simulink model "P3P_Grunert"  (R2023b)
settings: Solver=FixedStepDiscrete  StartTime=0.0  StopTime=0  RelTol=1e-3
values from neighbouring files (symbols this model uses):
  checkerSize = [5, 8]    [P3P_processVideo.m]
  checkerSquareLength = 31    [P3P_processVideo.m]
  I_current = I_allFrames(:,:,q)    [P3P_processVideo.m]
  K = [1107 0 960; 0 1107 540; 0 0 1]    [P3P_processVideo.m]
  x_pnts_i = round(x_pnts_i)    [P3P_processVideo.m]
undefined symbols (not defined in the file or in its folder): gray, Rec, SDTV, X_pnts_w
libraries: dspinverses x4, dspmathops x4, visiontextngfix x4, visionconversions x1, visionanalysis x1, dspvision x1, visionsources x1
(part 1 of 2)
settings Model: Creator=The MathWorks, Inc.  LastModifiedBy=alyss
settings DebuggingCC: ParameterPrecisionLossMsg=none  UnconnectedInputMsg=warning  UnconnectedOutputMsg=warning  UnconnectedLineMsg=warning  IntegerSaturationMsg=none
settings ModelReferenceCC: EnableRefExpFcnMdlSchedulingChecks=on
settings RTWCC: DLArmComputeVersion=19.05

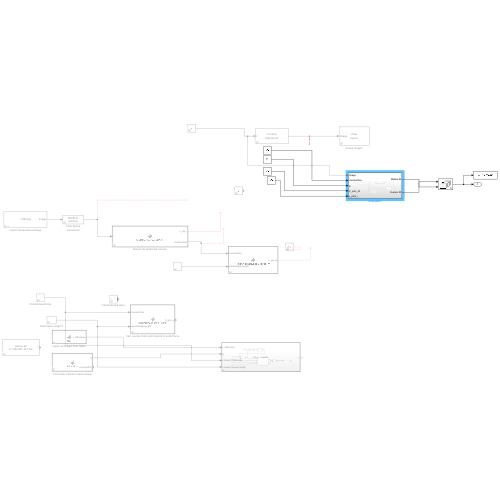
[thumbnail: Simulink's stored preview of the top-level diagram]
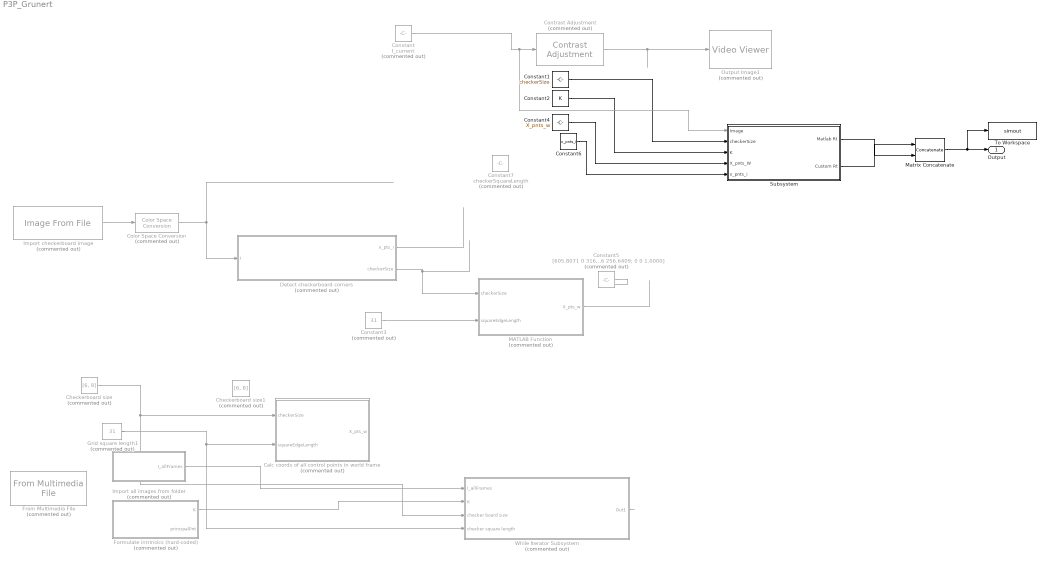
== system P3P_Grunert ==
  Calc coords of all control points in world frame : MATLAB Function  Commented=on  TreatAsAtomicUnit=on
  Checkerboard size : Constant  Commented=on  Value=[6, 8]
  Checkerboard size1 : Constant  Commented=on  Value=[6, 8]
  Color Space Conversion : visionconversions/Color Space  Conversion  Commented=on  conversion=Obsolete  conversionActive=R'G'B' to intensity  wp_str=D65  rec=Rec. 601 (SDTV)  sys=1125/60/2:1  imagePorts=One multidimensional signal
  Constant : Constant  Commented=on  Value=I_current
  Constant1 : Constant  Value=checkerSize
  Constant2 : Constant  Value=K
  Constant3 : Constant  Commented=on  Value=31
  Constant4 : Constant  Value=X_pnts_w
  Constant5 : Constant  Commented=on  Value=[605.8071 0 316.6903; 0 608.4646 256.6409; 0 0 1.0000]
  Constant6 : Constant  Value=x_pnts_i
  Constant7 : Constant  Commented=on  Value=checkerSquareLength
  Contrast Adjustment : visionanalysis/Contrast Adjustment  Commented=on  methodInputRange=Full input data range [min max]  rangeIn=[0 255]  fracSaturate=[1 1]  isBinNum=on  binNum=256  methodOutputRange=Full data type range  rangeOut=[0 255]  roundingMode=Floor  overflowMode=off  prod1Mode=Binary point scaling  prod1WordLength=32  prod1FracLength=16  prod2Mode=Binary point scaling  prod2WordLength=32  prod2FracLength=16
  Detect checkerboard corners : MATLAB Function  Commented=on  TreatAsAtomicUnit=on
  Formulate intrinsics (hard-coded) : MATLAB Function  Commented=on  TreatAsAtomicUnit=on
  From Multimedia File : dspvision/From Multimedia File  Commented=on  inputFilename=vipmen.avi  readRange=[1 Inf]  loop=on  numPlays=1  outputStreams=Video only  videoDataType=single  audioDataType=int16  inheritSampleTime=on  userDefinedSampleTime=1/30  noAudioOutput=off  isIntensityVideo=off  fourcc=Intensity  colorVideoFormat=One multidimensional signal  outputEOF=off  dataOrg=Column-major  audioFrameSize=1024  computeAudioFrameSize=off  outSamplingMode=Sample based
      settings: LibrarySourceBlock=visionsources/From Multimedia File
  Grid square length1 : Constant  Commented=on  Value=31
  Import all images from folder : MATLAB Function  Commented=on  TreatAsAtomicUnit=on
  Import checkerboard image : visionsources/Image From File  Tag=vipblks_nd  Commented=on  FileName=C:\Users\alyss\OneDrive - University of Cape Town\Code\MATLAB\PnP\Verification\-0160.jpg  Ts=inf  imagePorts=One multidimensional signal  OutPortLabels=R|G|B  ImageDataType=Inherit from input image  sdImageDataType=uint(8)  Signed=on  WordLength=16  FractionLengthMode=User-defined  FractionLength=15
  MATLAB Function : MATLAB Function  Commented=on  TreatAsAtomicUnit=on
  Matrix Concatenate : Concatenate  Mode=Multidimensional array  ConcatenateDimension=3
  Output Image1 : VideoViewer  Commented=on  colormapValue=gray(256)  FigPos=[1727 991 1362 617]
  Subsystem : Subsystem
  To Workspace : ToWorkspace  VariableName=simout  SampleTime=-1
  While Iterator Subsystem : Subsystem  Commented=on  TreatAsAtomicUnit=on
  Output : Outport
  wires:
  Import checkerboard image/1 -> Color Space Conversion/1
  Subsystem/1(Matlab Rt) -> Matrix Concatenate/2
  Subsystem/2(Custom Rt) -> Matrix Concatenate/1
  Matrix Concatenate/1 -> To Workspace/1, Output/1
  Formulate intrinsics (hard-coded)/1(K) -> While Iterator Subsystem/2(K)
  Grid square length1/1 -> Calc coords of all control points in world frame/2(squareEdgeLength), While Iterator Subsystem/4(checker square length)
  While Iterator Subsystem/1(Out1) -> ?
  Import all images from folder/1(I_allFrames) -> While Iterator Subsystem/1(I_allFrames)
  Constant3/1 -> MATLAB Function/2(squareEdgeLength)
  Checkerboard size/1 -> While Iterator Subsystem/3(checker board size), Calc coords of all control points in world frame/1(checkerSize)
  Constant4/1 -> Subsystem/4(X_pnts_W)
  Contrast Adjustment/1 -> Output Image1/1
  Constant1/1 -> Subsystem/2(checkerSize)
  Constant2/1 -> Subsystem/3(K)
  Color Space Conversion/1 -> Detect checkerboard corners/1(I)
  Constant/1 -> Subsystem/1(Image), Contrast Adjustment/1
  Constant6/1 -> Subsystem/5(x_pnts_i)
  Detect checkerboard corners/1(x_pts_i) -> ?
  Detect checkerboard corners/2(checkerSize) -> MATLAB Function/1(checkerSize)
  Constant5/1 -> ?
  MATLAB Function/1(X_pts_w) -> ?

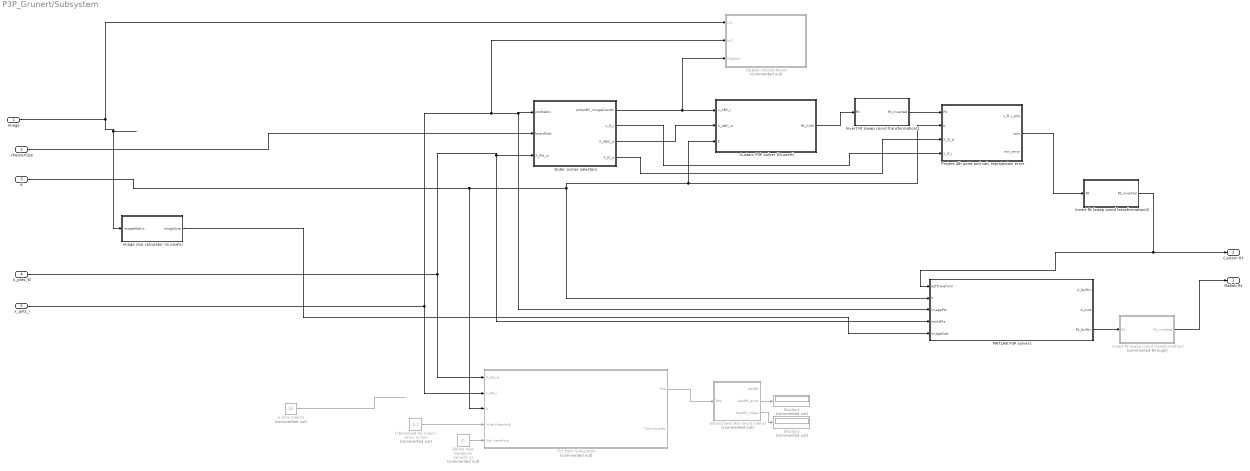
== system P3P_Grunert/Subsystem ==
  Image : Inport
  checkerSize : Inport  Port=2
  K : Inport  Port=3
  X_pnts_W : Inport  Port=4
  x_pnts_i : Inport  Port=5
  Custom P3P solver (Grunert) : Subsystem
  Define max iterations : Constant  Commented=on  Value=zeros(5,1)
  Display checkerboard : Subsystem  Commented=on
  Display4 : Display  Commented=on
  Display5 : Display  Commented=on
  Extract best Rte (most inliers) : MATLAB Function  Commented=on  TreatAsAtomicUnit=on
  For Each Subsystem : Subsystem  Commented=on  TreatAsAtomicUnit=on
  Image size calculator (in pixels) : MATLAB Function  TreatAsAtomicUnit=on
  Invert Rt (swap coord transformation) : MATLAB Function  Commented=through  TreatAsAtomicUnit=on
  Invert Rt (swap coord transformation)1 : MATLAB Function  TreatAsAtomicUnit=on
  Invert Rt (swap coord transformation)2 : MATLAB Function  TreatAsAtomicUnit=on
  MATLAB P3P solver1 : MATLAB Function  TreatAsAtomicUnit=on
  Outer corner selectors : Subsystem
  Project 4th point and calc reprojection error : MATLAB Function  TreatAsAtomicUnit=on
  n (min inliers) : Constant  Commented=on  Value=25
  t (threshold for inlier) - error in mm : Constant  Commented=on  Value=0.7
  Matlab Rt : Outport
  Custom Rt : Outport  Port=2
  wires:
  n (min inliers)/1 -> ?
  t (threshold for inlier) - error in mm/1 -> For Each Subsystem/4(Inlier threshold)
  Outer corner selectors/4(X_D_w) -> Project 4th point and calc reprojection error/3(X_D_w)
  Outer corner selectors/2(x_D_i) -> Project 4th point and calc reprojection error/4(x_D_i)
  x_pnts_i/1 -> MATLAB P3P solver1/3(imagePts), Outer corner selectors/1(pntMatrix), Display checkerboard/2(In2), For Each Subsystem/2(x_pts_i)
  Extract best Rte (most inliers)/2(bestRt_error) -> Display4/1
  Image/1 -> Image size calculator (in pixels)/1(imageMatrix), Display checkerboard/1(In1)
  X_pnts_W/1 -> MATLAB P3P solver1/4(worldPts), Outer corner selectors/3(X_Pts_w), For Each Subsystem/1(X_pts_w)
  For Each Subsystem/1(Rte) -> Extract best Rte (most inliers)/1(Rte)
  Outer corner selectors/3(X_ABC_w) -> Custom P3P solver (Grunert)/2(X_ABC_w)
  Extract best Rte (most inliers)/3(bestRt_inliers) -> Display5/1
  Image size calculator (in pixels)/1(imageSize) -> MATLAB P3P solver1/5(imageSize)
  K/1 -> For Each Subsystem/3(K), Project 4th point and calc reprojection error/2(K), Custom P3P solver (Grunert)/3(K), MATLAB P3P solver1/2(K)
  Define max iterations/1 -> For Each Subsystem/5(Vec iterations)
  Outer corner selectors/1(pntsABC_imageCoords) -> Display checkerboard/3(Outport), Custom P3P solver (Grunert)/1(x_ABC_i)
  checkerSize/1 -> Outer corner selectors/2(boardSize)
  MATLAB P3P solver1/3(Rt_builtin) -> Invert Rt (swap coord transformation)/1(Rt)
  Invert Rt (swap coord transformation)/1(Rt_inverted) -> Matlab Rt/1
  Invert Rt (swap coord transformation)2/1(Rt_inverted) -> MATLAB P3P solver1/1(estTransform), Custom Rt/1
  Custom P3P solver (Grunert)/1(Rt_C2W) -> Invert Rt (swap coord transformation)1/1(Rt)
  Invert Rt (swap coord transformation)1/1(Rt_inverted) -> Project 4th point and calc reprojection error/1(Rt)
  Project 4th point and calc reprojection error/2(soln) -> Invert Rt (swap coord transformation)2/1(Rt)

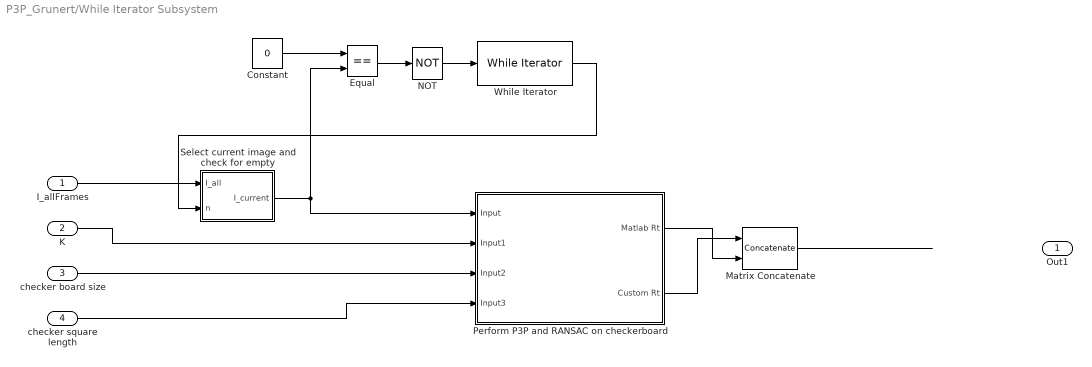
== system P3P_Grunert/While Iterator Subsystem ==
  I_allFrames : Inport
  K : Inport  Port=2
  checker board size : Inport  Port=3
  checker square length : Inport  Port=4
  Constant : Constant  Value=0
  Equal : RelationalOperator  Operator===  OutDataTypeStr=boolean  RndMeth=Simplest  InputSameDT=off
  Matrix Concatenate : Concatenate  Mode=Multidimensional array  ConcatenateDimension=3
  NOT : Logic  Operator=NOT  IconShape=distinctive  AllPortsSameDT=off  OutDataTypeStr=boolean
  Perform P3P and RANSAC on checkerboard : Subsystem  mask{intensityMatrix=[0 0; 0 0], checkerSize=[0, 0], K=[0 0 0; 0 0 0; 0 0 0], checkerSquareEdgeLength=0}
      mask prompts: intensityMatrix "2D matrix of pixel intensity values."; checkerSize "Number of squares in the checkerboard to be detected, specified as a 1D array [height, width]."; K "Camera intrinsic matrix, 3x3."; checkerSquareEdgeLength "Length of edge of one square in mm."
  Select current image and check for empty : MATLAB Function  TreatAsAtomicUnit=on
  While Iterator : WhileIterator  MaxIters=100  WhileBlockType=do-while  ShowIterationPort=on  OutputDataType=int16
  Out1 : Outport
  wires:
  I_allFrames/1 -> Select current image and check for empty/1(I_all)
  While Iterator/1 -> Select current image and check for empty/2(n)
  Constant/1 -> Equal/1
  NOT/1 -> While Iterator/1
  Equal/1 -> NOT/1
  Select current image and check for empty/1(I_current) -> Perform P3P and RANSAC on checkerboard/1(Input), Equal/2
  Matrix Concatenate/1 -> ?
  Perform P3P and RANSAC on checkerboard/2(Custom Rt) -> Matrix Concatenate/1
  K/1 -> Perform P3P and RANSAC on checkerboard/2(Input1)
  Perform P3P and RANSAC on checkerboard/1(Matlab Rt) -> Matrix Concatenate/2
  checker square length/1 -> Perform P3P and RANSAC on checkerboard/4(Input3)
  checker board size/1 -> Perform P3P and RANSAC on checkerboard/3(Input2)

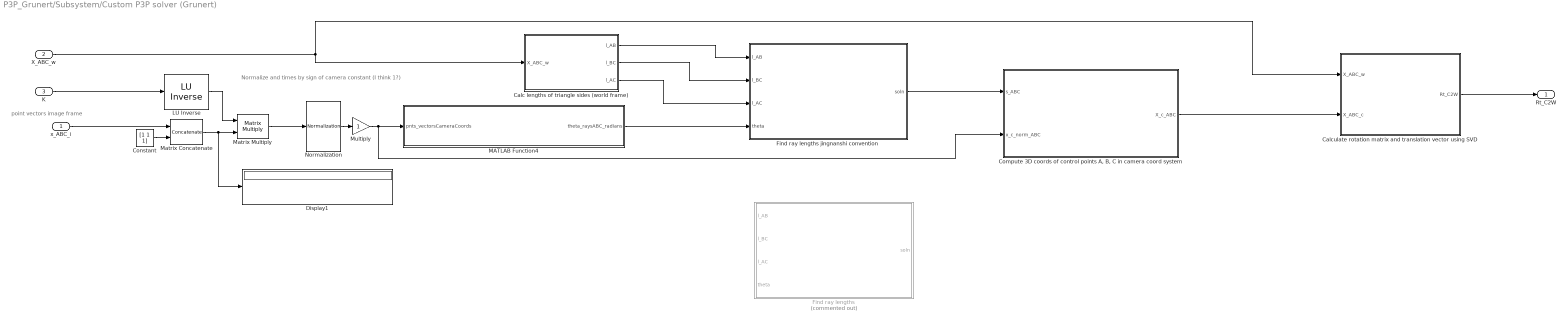
== system P3P_Grunert/Subsystem/Custom P3P solver (Grunert) ==
  note: point vectors image frame
  note: Normalize and times by sign of camera constant (I think 1?)
  x_ABC_i : Inport
  X_ABC_w : Inport  Port=2
  K : Inport  Port=3
  " LU Inverse" : dspinverses/ LU Inverse
  Calc lengths of triangle sides (world frame) : MATLAB Function  TreatAsAtomicUnit=on
  Calculate rotation matrix and translation vector using SVD : MATLAB Function  TreatAsAtomicUnit=on
  "Compute 3D coords of control points A, B, C in camera coord system" : MATLAB Function  TreatAsAtomicUnit=on
  Constant : Constant  Value=[1 1 1]  VectorParams1D=off
  Display1 : Display
  Find ray lengths : MATLAB Function  Commented=on  TreatAsAtomicUnit=on
  Find ray lengths jingnanshi convention : MATLAB Function  TreatAsAtomicUnit=on
  MATLAB Function4 : MATLAB Function  TreatAsAtomicUnit=on
  Matrix Concatenate : Concatenate  Mode=Multidimensional array
  Matrix Multiply : Product  Multiplication=Matrix(*)
  Multiply : Gain
  Normalization : dspmathops/Normalization  NormType=2-norm  Bias=1e-10  NormOver=Each column  Dimension=1  roundingMode=Floor  overflowMode=off  accumDataTypeStr=Inherit: Same as product output  accumLastDataTypeStr=Inherit: Same as product output  outputDataTypeStr=Inherit: Same as product output  outputMin=[]  outputMax=[]  outputLastDataTypeStr=Inherit: Same as product output
  Rt_C2W : Outport
  wires:
  Multiply/1 -> "Compute 3D coords of control points A, B, C in camera coord system"/2(x_c_norm_ABC), MATLAB Function4/1(pnts_vectorsCameraCoords)
  Normalization/1 -> Multiply/1
  MATLAB Function4/1(theta_raysABC_radians) -> Find ray lengths jingnanshi convention/4(theta)
  "Compute 3D coords of control points A, B, C in camera coord system"/1(X_c_ABC) -> Calculate rotation matrix and translation vector using SVD/2(X_ABC_c)
  X_ABC_w/1 -> Calculate rotation matrix and translation vector using SVD/1(X_ABC_w), Calc lengths of triangle sides (world frame)/1(X_ABC_w)
  Calc lengths of triangle sides (world frame)/3(l_AC) -> Find ray lengths jingnanshi convention/3(l_AC)
  Calc lengths of triangle sides (world frame)/1(l_AB) -> Find ray lengths jingnanshi convention/1(l_AB)
  Calc lengths of triangle sides (world frame)/2(l_BC) -> Find ray lengths jingnanshi convention/2(l_BC)
  K/1 -> " LU Inverse"/1
  Find ray lengths jingnanshi convention/1(soln) -> "Compute 3D coords of control points A, B, C in camera coord system"/1(s_ABC)
  x_ABC_i/1 -> Matrix Concatenate/1
  Matrix Concatenate/1 -> Display1/1, Matrix Multiply/2
  " LU Inverse"/1 -> Matrix Multiply/1
  Matrix Multiply/1 -> Normalization/1
  Constant/1 -> Matrix Concatenate/2
  Calculate rotation matrix and translation vector using SVD/1(Rt_C2W) -> Rt_C2W/1

== system P3P_Grunert/Subsystem/Display checkerboard ==
  In1 : Inport
  In2 : Inport  Port=2
  Outport : Inport  Port=3
  Data Type Conversion : DataTypeConversion  OutDataTypeStr=int16  SaturateOnIntegerOverflow=off  RndMeth=Floor
  Data Type Conversion1 : DataTypeConversion  OutDataTypeStr=int16  SaturateOnIntegerOverflow=off  RndMeth=Floor
  Draw All Detected Corners1 : visiontextngfix/Draw Markers  shape=Circle  size=4  fill=on  fillClrSource=Specify via dialog  display=User-specified value  intensity=200  color=250  opacity=0.6  viewport=Entire image  antialiasing=off  inType=Obsolete  imagePorts=One multidimensional signal  roundingMode=Floor  overflowMode=off  memoryMode=Specify word length  memoryWordLength=16  memoryFracLength=15  prodOutputMode=Binary point scaling  prodOutputWordLength=32  prodOutputFracLength=14
  Insert Text : visiontextngfix/Insert Text  inputType=Obsolete  theText='%s'  getTextLocFrom=Input port  textLoc=[100 100]  getTextColorFrom=Specify via dialog  textColor=[0 255 0]  getTextIntensityFrom=Specify via dialog  textIntensity=1  getTextOpacityFrom=Specify via dialog  textOpacity=1.0  dummyVar2=0  dummyVar3=0  dummyVar4=0  imagePorts=One multidimensional signal  isInputTransposed=off  fontFace=LucidaSansRegular  dummyVar1=0  blockFontSize=60  antiAliased=on
  Output Image1 : VideoViewer  colormapValue=gray(256)  FigPos=[2 725 1362 615]
  Specify text variables : Constant  Value=uint8(['A' 0 'B' 0 'C'])
  Transpose : Math  Operator=transpose
  wires:
  Data Type Conversion/1 -> Draw All Detected Corners1/2
  Draw All Detected Corners1/1 -> Insert Text/1
  Specify text variables/1 -> Insert Text/2
  Transpose/1 -> Insert Text/3
  In1/1 -> Draw All Detected Corners1/1
  Insert Text/1 -> Output Image1/1
  Data Type Conversion1/1 -> Transpose/1
  Outport/1 -> Data Type Conversion1/1
  In2/1 -> Data Type Conversion/1

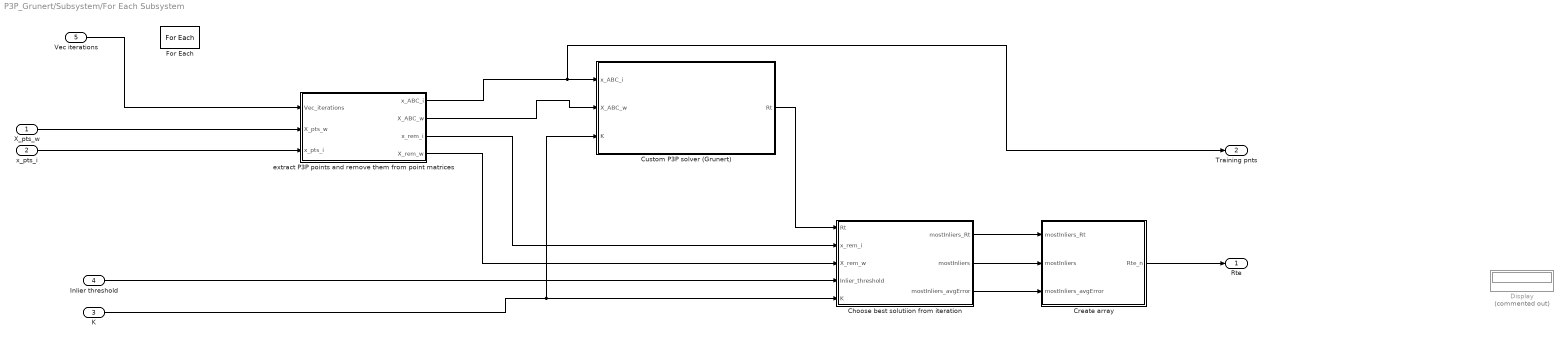
== system P3P_Grunert/Subsystem/For Each Subsystem ==
  X_pts_w : Inport
  x_pts_i : Inport  Port=2
  K : Inport  Port=3
  Inlier threshold : Inport  Port=4
  Vec iterations : Inport  Port=5  Partition=on  PartitionDimension=1  PartitionWidth=1  PartitionOffset=0
  Choose best solutiion from iteration : MATLAB Function  TreatAsAtomicUnit=on
  Create array : MATLAB Function  TreatAsAtomicUnit=on
  Custom P3P solver (Grunert) : Subsystem
  Display : Display  Commented=on
  For Each : ForEach  DisableCoverage=on
  extract P3P points and remove them from point matrices : MATLAB Function  TreatAsAtomicUnit=on
  Rte : Outport  ConcatenationDimension=3
  Training pnts : Outport  Port=2  ConcatenationDimension=2
  wires:
  Create array/1(Rte_n) -> Rte/1
  K/1 -> Custom P3P solver (Grunert)/3(K), Choose best solutiion from iteration/5(K)
  Choose best solutiion from iteration/2(mostInliers) -> Create array/2(mostInliers)
  Choose best solutiion from iteration/1(mostInliers_Rt) -> Create array/1(mostInliers_Rt)
  Inlier threshold/1 -> Choose best solutiion from iteration/4(Inlier_threshold)
  Custom P3P solver (Grunert)/1(Rt) -> Choose best solutiion from iteration/1(Rt)
  x_pts_i/1 -> extract P3P points and remove them from point matrices/3(x_pts_i)
  extract P3P points and remove them from point matrices/4(X_rem_w) -> Choose best solutiion from iteration/3(X_rem_w)
  extract P3P points and remove them from point matrices/1(x_ABC_i) -> Training pnts/1, Custom P3P solver (Grunert)/1(x_ABC_i)
  X_pts_w/1 -> extract P3P points and remove them from point matrices/2(X_pts_w)
  extract P3P points and remove them from point matrices/2(X_ABC_w) -> Custom P3P solver (Grunert)/2(X_ABC_w)
  extract P3P points and remove them from point matrices/3(x_rem_i) -> Choose best solutiion from iteration/2(x_rem_i)
  Choose best solutiion from iteration/3(mostInliers_avgError) -> Create array/3(mostInliers_avgError)
  Vec iterations/1 -> extract P3P points and remove them from point matrices/1(Vec_iterations)

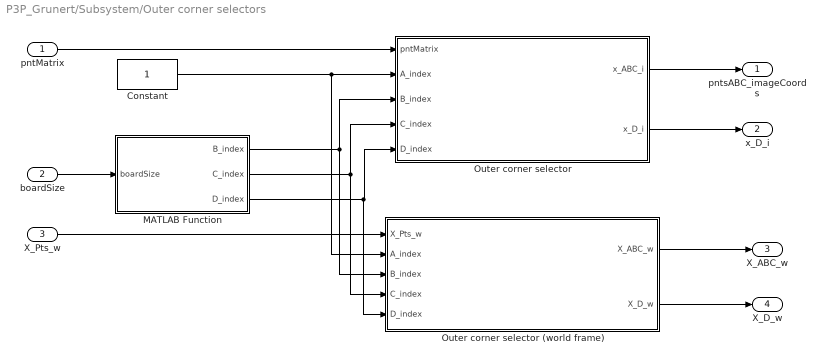
== system P3P_Grunert/Subsystem/Outer corner selectors ==
  pntMatrix : Inport
  boardSize : Inport  Port=2
  X_Pts_w : Inport  Port=3
  Constant : Constant
  MATLAB Function : MATLAB Function  TreatAsAtomicUnit=on
  Outer corner selector : MATLAB Function  TreatAsAtomicUnit=on
  Outer corner selector (world frame) : MATLAB Function  TreatAsAtomicUnit=on
  pntsABC_imageCoords : Outport
  x_D_i : Outport  Port=2
  X_ABC_w : Outport  Port=3
  X_D_w : Outport  Port=4
  wires:
  Outer corner selector/2(x_D_i) -> x_D_i/1
  Outer corner selector (world frame)/1(X_ABC_w) -> X_ABC_w/1
  Outer corner selector/1(x_ABC_i) -> pntsABC_imageCoords/1
  Outer corner selector (world frame)/2(X_D_w) -> X_D_w/1
  boardSize/1 -> MATLAB Function/1(boardSize)
  pntMatrix/1 -> Outer corner selector/1(pntMatrix)
  X_Pts_w/1 -> Outer corner selector (world frame)/1(X_Pts_w)
  Constant/1 -> Outer corner selector (world frame)/2(A_index), Outer corner selector/2(A_index)
  MATLAB Function/1(B_index) -> Outer corner selector/3(B_index), Outer corner selector (world frame)/3(B_index)
  MATLAB Function/2(C_index) -> Outer corner selector/4(C_index), Outer corner selector (world frame)/4(C_index)
  MATLAB Function/3(D_index) -> Outer corner selector (world frame)/5(D_index), Outer corner selector/5(D_index)

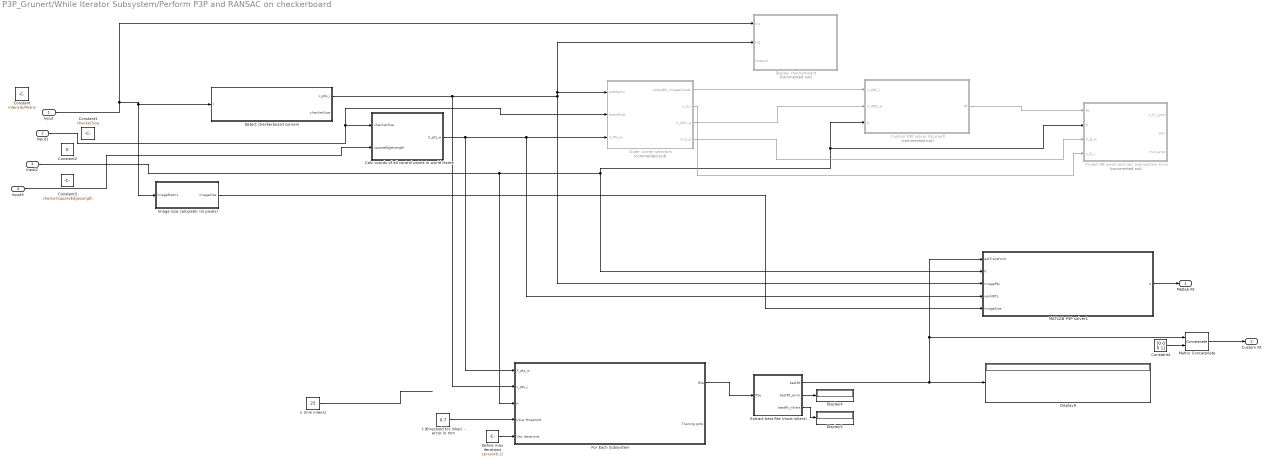
== system P3P_Grunert/While Iterator Subsystem/Perform P3P and RANSAC on checkerboard ==
  Input : Inport
  Input1 : Inport  Port=2
  Input2 : Inport  Port=3
  Input3 : Inport  Port=4
  Calc coords of all control points in world frame : MATLAB Function  TreatAsAtomicUnit=on
  Constant : Constant  Value=intensityMatrix
  Constant1 : Constant  Value=checkerSize
  Constant2 : Constant  Value=K
  Constant3 : Constant  Value=checkerSquareEdgeLength
  Constant4 : Constant  Value=[0 0 0 1]  VectorParams1D=off
  Custom P3P solver (Grunert) : Subsystem  Commented=on
  Define max iterations : Constant  Value=zeros(40,1)
  Detect checkerboard corners : MATLAB Function  TreatAsAtomicUnit=on
  Display checkerboard : Subsystem  Commented=on
  Display4 : Display
  Display5 : Display
  Display6 : Display
  Extract best Rte (most inliers) : MATLAB Function  TreatAsAtomicUnit=on
  For Each Subsystem : Subsystem  TreatAsAtomicUnit=on
  Image size calculator (in pixels) : MATLAB Function  TreatAsAtomicUnit=on
  MATLAB P3P solver1 : MATLAB Function  TreatAsAtomicUnit=on
  Matrix Concatenate : Concatenate  Mode=Multidimensional array
  Outer corner selectors : Subsystem  Commented=on
  Project 4th point and calc reprojection error : MATLAB Function  Commented=on  TreatAsAtomicUnit=on
  n (min inliers) : Constant  Value=25
  t (threshold for inlier) - error in mm : Constant  Value=0.7
  Matlab Rt : Outport
  Custom Rt : Outport  Port=2
  wires:
  Input1/1 -> Outer corner selectors/2(boardSize), Calc coords of all control points in world frame/1(checkerSize)
  Outer corner selectors/3(X_ABC_w) -> Custom P3P solver (Grunert)/2(X_ABC_w)
  Calc coords of all control points in world frame/1(X_pts_w) -> For Each Subsystem/1(X_pts_w), MATLAB P3P solver1/4(worldPts), Outer corner selectors/3(X_Pts_w)
  Outer corner selectors/1(pntsABC_imageCoords) -> Custom P3P solver (Grunert)/1(x_ABC_i)
  Input2/1 -> For Each Subsystem/3(K), Project 4th point and calc reprojection error/2(K), Custom P3P solver (Grunert)/3(K), MATLAB P3P solver1/2(K)
  Detect checkerboard corners/1(x_pts_i) -> Display checkerboard/2(In2), Outer corner selectors/1(pntMatrix), MATLAB P3P solver1/3(imagePts), For Each Subsystem/2(x_pts_i)
  Extract best Rte (most inliers)/3(bestRt_inliers) -> Display5/1
  For Each Subsystem/1(Rte) -> Extract best Rte (most inliers)/1(Rte)
  Image size calculator (in pixels)/1(imageSize) -> MATLAB P3P solver1/5(imageSize)
  Extract best Rte (most inliers)/1(bestRt) -> MATLAB P3P solver1/1(estTransform), Matrix Concatenate/1, Display6/1
  Define max iterations/1 -> For Each Subsystem/5(Vec iterations)
  Custom P3P solver (Grunert)/1(Rt) -> Project 4th point and calc reprojection error/1(Rt)
  t (threshold for inlier) - error in mm/1 -> For Each Subsystem/4(Inlier threshold)
  Input/1 -> Display checkerboard/1(In1), Image size calculator (in pixels)/1(imageMatrix), Detect checkerboard corners/1(I)
  Extract best Rte (most inliers)/2(bestRt_error) -> Display4/1
  Outer corner selectors/4(X_D_w) -> Project 4th point and calc reprojection error/3(X_D_w)
  Outer corner selectors/2(x_D_i) -> Project 4th point and calc reprojection error/4(x_D_i)
  Input3/1 -> Calc coords of all control points in world frame/2(squareEdgeLength)
  MATLAB P3P solver1/1(A) -> Matlab Rt/1
  n (min inliers)/1 -> ?
  Constant4/1 -> Matrix Concatenate/2
  Matrix Concatenate/1 -> Custom Rt/1

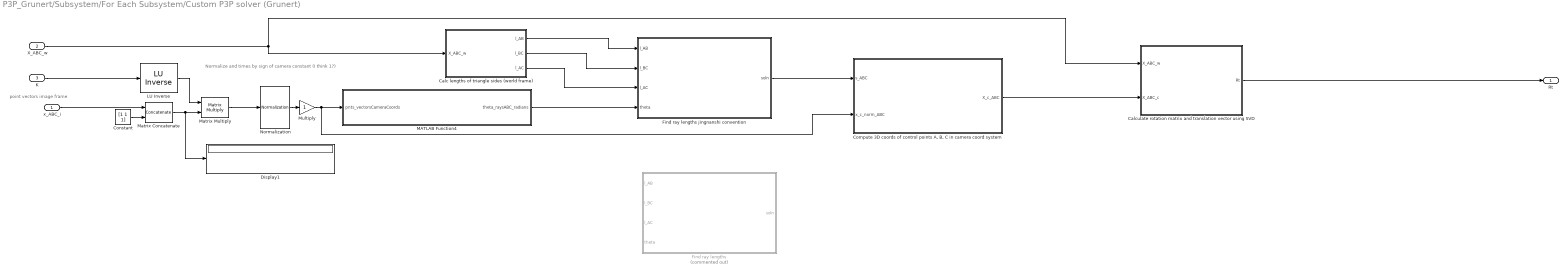
== system P3P_Grunert/Subsystem/For Each Subsystem/Custom P3P solver (Grunert) ==
  note: point vectors image frame
  note: Normalize and times by sign of camera constant (I think 1?)
  x_ABC_i : Inport
  X_ABC_w : Inport  Port=2
  K : Inport  Port=3
  " LU Inverse" : dspinverses/ LU Inverse
  Calc lengths of triangle sides (world frame) : MATLAB Function  TreatAsAtomicUnit=on
  Calculate rotation matrix and translation vector using SVD : MATLAB Function  TreatAsAtomicUnit=on
  "Compute 3D coords of control points A, B, C in camera coord system" : MATLAB Function  TreatAsAtomicUnit=on
  Constant : Constant  Value=[1 1 1]  VectorParams1D=off
  Display1 : Display
  Find ray lengths : MATLAB Function  Commented=on  TreatAsAtomicUnit=on
  Find ray lengths jingnanshi convention : MATLAB Function  TreatAsAtomicUnit=on
  MATLAB Function4 : MATLAB Function  TreatAsAtomicUnit=on
  Matrix Concatenate : Concatenate  Mode=Multidimensional array
  Matrix Multiply : Product  Multiplication=Matrix(*)
  Multiply : Gain
  Normalization : dspmathops/Normalization  NormType=2-norm  Bias=1e-10  NormOver=Each column  Dimension=1  roundingMode=Floor  overflowMode=off  accumDataTypeStr=Inherit: Same as product output  accumLastDataTypeStr=Inherit: Same as product output  outputDataTypeStr=Inherit: Same as product output  outputMin=[]  outputMax=[]  outputLastDataTypeStr=Inherit: Same as product output
  Rt : Outport
  wires:
  Multiply/1 -> "Compute 3D coords of control points A, B, C in camera coord system"/2(x_c_norm_ABC), MATLAB Function4/1(pnts_vectorsCameraCoords)
  Normalization/1 -> Multiply/1
  MATLAB Function4/1(theta_raysABC_radians) -> Find ray lengths jingnanshi convention/4(theta)
  "Compute 3D coords of control points A, B, C in camera coord system"/1(X_c_ABC) -> Calculate rotation matrix and translation vector using SVD/2(X_ABC_c)
  X_ABC_w/1 -> Calculate rotation matrix and translation vector using SVD/1(X_ABC_w), Calc lengths of triangle sides (world frame)/1(X_ABC_w)
  Calc lengths of triangle sides (world frame)/3(l_AC) -> Find ray lengths jingnanshi convention/3(l_AC)
  Calc lengths of triangle sides (world frame)/1(l_AB) -> Find ray lengths jingnanshi convention/1(l_AB)
  Calc lengths of triangle sides (world frame)/2(l_BC) -> Find ray lengths jingnanshi convention/2(l_BC)
  K/1 -> " LU Inverse"/1
  Find ray lengths jingnanshi convention/1(soln) -> "Compute 3D coords of control points A, B, C in camera coord system"/1(s_ABC)
  x_ABC_i/1 -> Matrix Concatenate/1
  Matrix Concatenate/1 -> Display1/1, Matrix Multiply/2
  " LU Inverse"/1 -> Matrix Multiply/1
  Matrix Multiply/1 -> Normalization/1
  Constant/1 -> Matrix Concatenate/2
  Calculate rotation matrix and translation vector using SVD/1(Rt) -> Rt/1

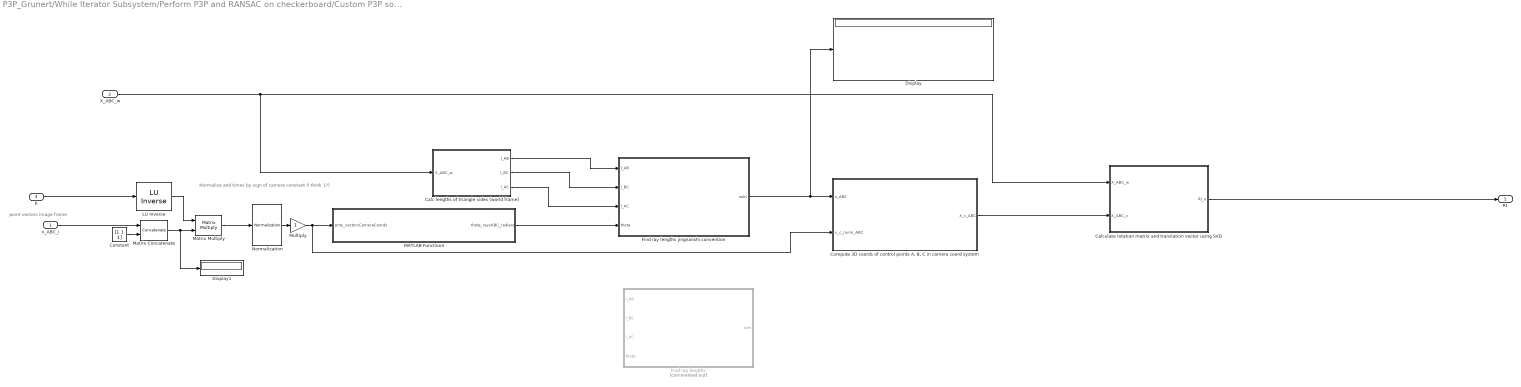
== system P3P_Grunert/While Iterator Subsystem/Perform P3P and RANSAC on checkerboard/Custom P3P solver (Grunert) ==
  note: point vectors image frame
  note: Normalize and times by sign of camera constant (I think 1?)
  x_ABC_i : Inport
  X_ABC_w : Inport  Port=2
  K : Inport  Port=3
  " LU Inverse" : dspinverses/ LU Inverse
  Calc lengths of triangle sides (world frame) : MATLAB Function  TreatAsAtomicUnit=on
  Calculate rotation matrix and translation vector using SVD : MATLAB Function  TreatAsAtomicUnit=on
  "Compute 3D coords of control points A, B, C in camera coord system" : MATLAB Function  TreatAsAtomicUnit=on
  Constant : Constant  Value=[1 1 1]  VectorParams1D=off
  Display : Display
  Display1 : Display
  Find ray lengths : MATLAB Function  Commented=on  TreatAsAtomicUnit=on
  Find ray lengths jingnanshi convention : MATLAB Function  TreatAsAtomicUnit=on
  MATLAB Function4 : MATLAB Function  TreatAsAtomicUnit=on
  Matrix Concatenate : Concatenate  Mode=Multidimensional array
  Matrix Multiply : Product  Multiplication=Matrix(*)
  Multiply : Gain
  Normalization : dspmathops/Normalization  NormType=2-norm  Bias=1e-10  NormOver=Each column  Dimension=1  roundingMode=Floor  overflowMode=off  accumDataTypeStr=Inherit: Same as product output  accumLastDataTypeStr=Inherit: Same as product output  outputDataTypeStr=Inherit: Same as product output  outputMin=[]  outputMax=[]  outputLastDataTypeStr=Inherit: Same as product output
  Rt : Outport
  wires:
  Multiply/1 -> "Compute 3D coords of control points A, B, C in camera coord system"/2(x_c_norm_ABC), MATLAB Function4/1(pnts_vectorsCameraCoords)
  Normalization/1 -> Multiply/1
  MATLAB Function4/1(theta_raysABC_radians) -> Find ray lengths jingnanshi convention/4(theta)
  "Compute 3D coords of control points A, B, C in camera coord system"/1(X_c_ABC) -> Calculate rotation matrix and translation vector using SVD/2(X_ABC_c)
  X_ABC_w/1 -> Calc lengths of triangle sides (world frame)/1(X_ABC_w), Calculate rotation matrix and translation vector using SVD/1(X_ABC_w)
  Calc lengths of triangle sides (world frame)/3(l_AC) -> Find ray lengths jingnanshi convention/3(l_AC)
  Calc lengths of triangle sides (world frame)/1(l_AB) -> Find ray lengths jingnanshi convention/1(l_AB)
  Calc lengths of triangle sides (world frame)/2(l_BC) -> Find ray lengths jingnanshi convention/2(l_BC)
  K/1 -> " LU Inverse"/1
  Find ray lengths jingnanshi convention/1(soln) -> "Compute 3D coords of control points A, B, C in camera coord system"/1(s_ABC), Display/1
  x_ABC_i/1 -> Matrix Concatenate/1
  Matrix Concatenate/1 -> Display1/1, Matrix Multiply/2
  " LU Inverse"/1 -> Matrix Multiply/1
  Matrix Multiply/1 -> Normalization/1
  Constant/1 -> Matrix Concatenate/2
  Calculate rotation matrix and translation vector using SVD/1(Rt_o) -> Rt/1

== system P3P_Grunert/While Iterator Subsystem/Perform P3P and RANSAC on checkerboard/Display checkerboard ==
  In1 : Inport
  In2 : Inport  Port=2
  Outport : Inport  Port=3
  Data Type Conversion : DataTypeConversion  OutDataTypeStr=int16  SaturateOnIntegerOverflow=off  RndMeth=Floor
  Data Type Conversion1 : DataTypeConversion  OutDataTypeStr=int16  SaturateOnIntegerOverflow=off  RndMeth=Floor
  Draw All Detected Corners1 : visiontextngfix/Draw Markers  shape=Circle  size=9  fill=on  fillClrSource=Specify via dialog  display=User-specified value  intensity=200  color=[250 0 0]  opacity=0.6  viewport=Entire image  antialiasing=off  inType=Obsolete  imagePorts=One multidimensional signal  roundingMode=Floor  overflowMode=off  memoryMode=Specify word length  memoryWordLength=16  memoryFracLength=15  prodOutputMode=Binary point scaling  prodOutputWordLength=32  prodOutputFracLength=14
  Insert Text : visiontextngfix/Insert Text  inputType=Obsolete  theText='%s'  getTextLocFrom=Input port  textLoc=[100 100]  getTextColorFrom=Specify via dialog  textColor=[0 255 0]  getTextIntensityFrom=Specify via dialog  textIntensity=1  getTextOpacityFrom=Specify via dialog  textOpacity=1.0  dummyVar2=0  dummyVar3=0  dummyVar4=0  imagePorts=One multidimensional signal  isInputTransposed=off  fontFace=LucidaSansRegular  dummyVar1=0  blockFontSize=60  antiAliased=on
  Output Image1 : VideoViewer  colormapValue=gray(256)  FigPos=[2313 1141 833 686]
  Specify text variables : Constant  Value=uint8(['A' 0 'B' 0 'C'])
  Transpose : Math  Operator=transpose
  wires:
  Data Type Conversion/1 -> Draw All Detected Corners1/2
  Draw All Detected Corners1/1 -> Insert Text/1
  Specify text variables/1 -> Insert Text/2
  Transpose/1 -> Insert Text/3
  In1/1 -> Draw All Detected Corners1/1
  Insert Text/1 -> Output Image1/1
  Data Type Conversion1/1 -> Transpose/1
  Outport/1 -> Data Type Conversion1/1
  In2/1 -> Data Type Conversion/1

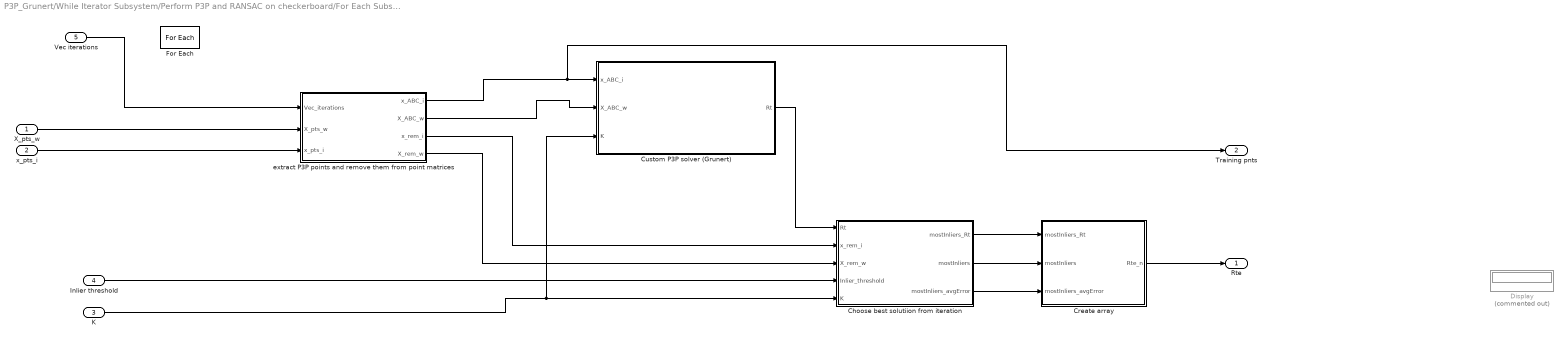
== system P3P_Grunert/While Iterator Subsystem/Perform P3P and RANSAC on checkerboard/For Each Subsystem ==
  X_pts_w : Inport
  x_pts_i : Inport  Port=2
  K : Inport  Port=3
  Inlier threshold : Inport  Port=4
  Vec iterations : Inport  Port=5  Partition=on  PartitionDimension=1  PartitionWidth=1  PartitionOffset=0
  Choose best solutiion from iteration : MATLAB Function  TreatAsAtomicUnit=on
  Create array : MATLAB Function  TreatAsAtomicUnit=on
  Custom P3P solver (Grunert) : Subsystem
  Display : Display  Commented=on
  For Each : ForEach  DisableCoverage=on
  extract P3P points and remove them from point matrices : MATLAB Function  TreatAsAtomicUnit=on
  Rte : Outport  ConcatenationDimension=3
  Training pnts : Outport  Port=2  ConcatenationDimension=2
  wires:
  Create array/1(Rte_n) -> Rte/1
  K/1 -> Custom P3P solver (Grunert)/3(K), Choose best solutiion from iteration/5(K)
  Choose best solutiion from iteration/2(mostInliers) -> Create array/2(mostInliers)
  Choose best solutiion from iteration/1(mostInliers_Rt) -> Create array/1(mostInliers_Rt)
  Inlier threshold/1 -> Choose best solutiion from iteration/4(Inlier_threshold)
  Custom P3P solver (Grunert)/1(Rt) -> Choose best solutiion from iteration/1(Rt)
  x_pts_i/1 -> extract P3P points and remove them from point matrices/3(x_pts_i)
  extract P3P points and remove them from point matrices/4(X_rem_w) -> Choose best solutiion from iteration/3(X_rem_w)
  extract P3P points and remove them from point matrices/1(x_ABC_i) -> Training pnts/1, Custom P3P solver (Grunert)/1(x_ABC_i)
  X_pts_w/1 -> extract P3P points and remove them from point matrices/2(X_pts_w)
  extract P3P points and remove them from point matrices/2(X_ABC_w) -> Custom P3P solver (Grunert)/2(X_ABC_w)
  extract P3P points and remove them from point matrices/3(x_rem_i) -> Choose best solutiion from iteration/2(x_rem_i)
  Choose best solutiion from iteration/3(mostInliers_avgError) -> Create array/3(mostInliers_avgError)
  Vec iterations/1 -> extract P3P points and remove them from point matrices/1(Vec_iterations)

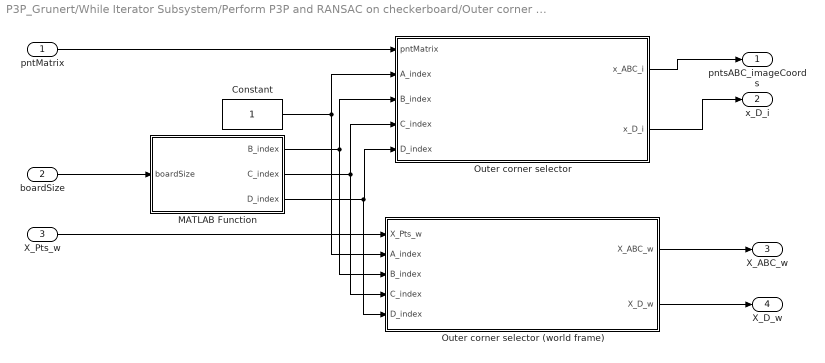
== system P3P_Grunert/While Iterator Subsystem/Perform P3P and RANSAC on checkerboard/Outer corner selectors ==
  pntMatrix : Inport
  boardSize : Inport  Port=2
  X_Pts_w : Inport  Port=3
  Constant : Constant
  MATLAB Function : MATLAB Function  TreatAsAtomicUnit=on
  Outer corner selector : MATLAB Function  TreatAsAtomicUnit=on
  Outer corner selector (world frame) : MATLAB Function  TreatAsAtomicUnit=on
  pntsABC_imageCoords : Outport
  x_D_i : Outport  Port=2
  X_ABC_w : Outport  Port=3
  X_D_w : Outport  Port=4
  wires:
  Outer corner selector/2(x_D_i) -> x_D_i/1
  Outer corner selector (world frame)/1(X_ABC_w) -> X_ABC_w/1
  Outer corner selector/1(x_ABC_i) -> pntsABC_imageCoords/1
  Outer corner selector (world frame)/2(X_D_w) -> X_D_w/1
  boardSize/1 -> MATLAB Function/1(boardSize)
  pntMatrix/1 -> Outer corner selector/1(pntMatrix)
  X_Pts_w/1 -> Outer corner selector (world frame)/1(X_Pts_w)
  Constant/1 -> Outer corner selector/2(A_index), Outer corner selector (world frame)/2(A_index)
  MATLAB Function/1(B_index) -> Outer corner selector/3(B_index), Outer corner selector (world frame)/3(B_index)
  MATLAB Function/2(C_index) -> Outer corner selector/4(C_index), Outer corner selector (world frame)/4(C_index)
  MATLAB Function/3(D_index) -> Outer corner selector (world frame)/5(D_index), Outer corner selector/5(D_index)

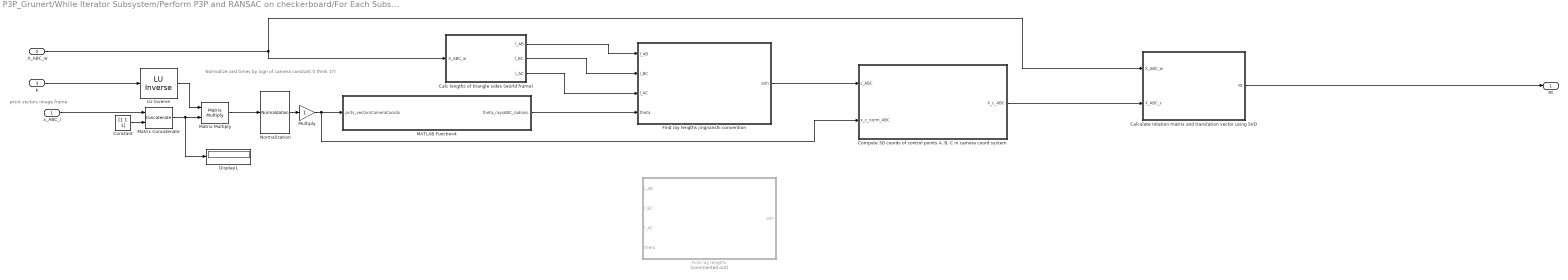
== system P3P_Grunert/While Iterator Subsystem/Perform P3P and RANSAC on checkerboard/For Each Subsystem/Custom P3P solver (Grunert) ==
  note: point vectors image frame
  note: Normalize and times by sign of camera constant (I think 1?)
  x_ABC_i : Inport
  X_ABC_w : Inport  Port=2
  K : Inport  Port=3
  " LU Inverse" : dspinverses/ LU Inverse
  Calc lengths of triangle sides (world frame) : MATLAB Function  TreatAsAtomicUnit=on
  Calculate rotation matrix and translation vector using SVD : MATLAB Function  TreatAsAtomicUnit=on
  "Compute 3D coords of control points A, B, C in camera coord system" : MATLAB Function  TreatAsAtomicUnit=on
  Constant : Constant  Value=[1 1 1]  VectorParams1D=off
  Display1 : Display
  Find ray lengths : MATLAB Function  Commented=on  TreatAsAtomicUnit=on
  Find ray lengths jingnanshi convention : MATLAB Function  TreatAsAtomicUnit=on
  MATLAB Function4 : MATLAB Function  TreatAsAtomicUnit=on
  Matrix Concatenate : Concatenate  Mode=Multidimensional array
  Matrix Multiply : Product  Multiplication=Matrix(*)
  Multiply : Gain
  Normalization : dspmathops/Normalization  NormType=2-norm  Bias=1e-10  NormOver=Each column  Dimension=1  roundingMode=Floor  overflowMode=off  accumDataTypeStr=Inherit: Same as product output  accumLastDataTypeStr=Inherit: Same as product output  outputDataTypeStr=Inherit: Same as product output  outputMin=[]  outputMax=[]  outputLastDataTypeStr=Inherit: Same as product output
  Rt : Outport
  wires:
  Multiply/1 -> "Compute 3D coords of control points A, B, C in camera coord system"/2(x_c_norm_ABC), MATLAB Function4/1(pnts_vectorsCameraCoords)
  Normalization/1 -> Multiply/1
  MATLAB Function4/1(theta_raysABC_radians) -> Find ray lengths jingnanshi convention/4(theta)
  "Compute 3D coords of control points A, B, C in camera coord system"/1(X_c_ABC) -> Calculate rotation matrix and translation vector using SVD/2(X_ABC_c)
  X_ABC_w/1 -> Calculate rotation matrix and translation vector using SVD/1(X_ABC_w), Calc lengths of triangle sides (world frame)/1(X_ABC_w)
  Calc lengths of triangle sides (world frame)/3(l_AC) -> Find ray lengths jingnanshi convention/3(l_AC)
  Calc lengths of triangle sides (world frame)/1(l_AB) -> Find ray lengths jingnanshi convention/1(l_AB)
  Calc lengths of triangle sides (world frame)/2(l_BC) -> Find ray lengths jingnanshi convention/2(l_BC)
  K/1 -> " LU Inverse"/1
  Find ray lengths jingnanshi convention/1(soln) -> "Compute 3D coords of control points A, B, C in camera coord system"/1(s_ABC)
  x_ABC_i/1 -> Matrix Concatenate/1
  Matrix Concatenate/1 -> Display1/1, Matrix Multiply/2
  " LU Inverse"/1 -> Matrix Multiply/1
  Matrix Multiply/1 -> Normalization/1
  Constant/1 -> Matrix Concatenate/2
  Calculate rotation matrix and translation vector using SVD/1(Rt) -> Rt/1

== matlab function P3P_Grunert/Import all images from folder ==
  data: I_allFrames output
function I_allFrames = fcn()

files_ds = fileDatastore(fullfile(uigetdir), 'ReadFcn', @importdata, "FileExtensions",".jpg");
allFileNames = fds.Files;
numFiles = length(allFileNames);

I_allFrames = zeros(2,2,numFiles);


%Loop to read all image files and put them into a multidim array
for n=1: numFiles

    I_colour = imread(allFileNames(n));
    I_gray = rgb2gray(I_colour);
    I_allFrames = I_gray(:,:,n);
end

== matlab function P3P_Grunert/While Iterator Subsystem/Select current image and check for empty ==
  data: I_all input; I_current output; n input
function I_current = fcn(I_all, n)

if isempty(I_all(:,:,n))
    I_current = 0;
else
    I_current = (I_all(:,:,n));
end

== matlab function P3P_Grunert/While Iterator Subsystem/Perform P3P and RANSAC on checkerboard/Calc coords of all control points in world frame ==
  data: X_pts_w output size=[60, 3]; checkerSize input; squareEdgeLength input
function X_pts_w = calcPtoPLengths_world(checkerSize, squareEdgeLength)
    
    boardWidth = checkerSize(2);
    boardHeight = checkerSize(1);
    X_pts_w = zeros((boardWidth-1)*(boardHeight-1), 3);

    %for each column
    for c=1 : boardWidth-1
        for r = 1: boardHeight-1
            x = (c-1)*squareEdgeLength;
            y = (r-1)*squareEdgeLength;
            z = 0;
            X_pts_w(  (((c-1)*(boardHeight-1)) + r), 1) = x;
            X_pts_w(  (((c-1)*(boardHeight-1)) + r), 2) = y;
            X_pts_w(  (((c-1)*(boardHeight-1)) + r), 3) = z;
        end
    end

== matlab function P3P_Grunert/While Iterator Subsystem/Perform P3P and RANSAC on checkerboard/Custom P3P solver (Grunert)/Calc lengths of triangle sides (world frame) ==
  data: X_ABC_w input; l_AB output; l_BC output; l_AC output
function [l_AB, l_BC, l_AC]= fcn(X_ABC_w)

l_AB = norm(X_ABC_w(:,1)-X_ABC_w(:,2));
l_AC = norm(X_ABC_w(:,1)-X_ABC_w(:,3));
l_BC = norm(X_ABC_w(:,2)-X_ABC_w(:,3));

== matlab function P3P_Grunert/While Iterator Subsystem/Perform P3P and RANSAC on checkerboard/Custom P3P solver (Grunert)/Calculate rotation matrix and translation vector using SVD ==
  data: X_ABC_w input; Rt_o output size=[3,4,4]; X_ABC_c input
function Rt_o = fcn(X_ABC_w, X_ABC_c)

%We have 3 points in the world frame and in the camera frame. Now we need 
%to find the rotation and translation matrices that would convert one to 
%the other.
%This is the classic Procrustes problem, which we can solve using singular 
%value decomposition. We will end up with one rotation matrix and one
%translation vector for each of the possible sets of coordinates. 

 R = zeros(3,3,4);
 t = zeros(3,4);
 Rt_o = zeros(3,4,4);

 P = X_ABC_w;
 %Find the mean of the columns (i.e. the centroid of the shape)
 P_centroid = mean(P,2);
 %Centre each vector
 Q = P - P_centroid;

%for each possible solution
for i=1: size(X_ABC_c, 3)

    %Condition each vector as above
    P_dash =  X_ABC_c(:, :, i);
    P_dash_centroid = mean(P_dash, 2);
    Q_dash = P_dash - P_dash_centroid;
    
    %Find the covariance matrix
    H = Q_dash * transpose(Q);

    %Perform SVD (singular value decomposition)
    [U, S, V] = svd(H);

    %Calculate rotation matrix
    R(:,:,i) = U * transpose(V);
    %Correct sign if needed
    if det(R(:,:,i))<0
        U(:,end) = U(:,end) * (-1);
        %and recompute R
        R(:, :, i) = U * transpose(V);
    end

    %Calculate the translation vector:
    t(:, i) = P_dash_centroid - R(:, :, i)*P_centroid;

    Rt_o(:,:, i)= [R(:,:,i) t(:, i)];

end

== matlab function P3P_Grunert/While Iterator Subsystem/Perform P3P and RANSAC on checkerboard/Custom P3P solver (Grunert)/Compute 3D coords of control points A, B, C in camera coord system ==
  data: s_ABC input; X_c_ABC output size=[3,3,4]; x_c_norm_ABC input
function X_c_ABC = fcn(s_ABC, x_c_norm_ABC)
    X_c_ABC = zeros(3,3,4);


    %For each combination of possible lengths
    for n=1:size(s_ABC, 1)
        %Get the vector between the camera and the point by multiplying
        %each element of the (unit) direction vector with the associated
        %ray length from the solution. 
        %The solution takes the form: [s_A1 s_B1 s_C1; s_A2 sB2...].
        %The direction vectors take the form: [xA xB xC; yA yB...].
        X_c_ABC(:, 1, n) = s_ABC(n, 1) * x_c_norm_ABC(:, 1);
        X_c_ABC(:, 2, n) = s_ABC(n, 2) * x_c_norm_ABC(:, 2);
        X_c_ABC(:, 3, n) = s_ABC(n, 3) * x_c_norm_ABC(:, 3);
    end

== matlab function P3P_Grunert/While Iterator Subsystem/Perform P3P and RANSAC on checkerboard/Custom P3P solver (Grunert)/Find ray lengths ==
  data: l_AB input; soln output size=[4, 3]; l_BC input; l_AC input; theta input
function soln = fcn(l_AB, l_BC, l_AC, theta)

soln = zeros(4, 3);


%Calculate polynomial coefficients
a = l_BC;
b = l_AC;
c = l_AB;

gamma = theta(3); %theta_AC
alpha = theta(2); %theta_BC
beta = theta(1); %theta_AB


a2minc2ovb2 =  (a^2 - c^2) / b^2 ;
a2plusc2ovb2 =  (a^2 + c^2) / b^2; 


A0 = (1 + a2minc2ovb2)^2   -   4*((a*cos(gamma)/b)^2);
A1 = - a2minc2ovb2 * (1 + a2minc2ovb2) * cos(beta)     +    2 * ((a * cos(gamma) /  b)^2) * cos (beta)     -     (1 - a2plusc2ovb2) * cos(alpha) * cos(gamma);
A1 = 4 * A1;
A2 = a2minc2ovb2^2   -   1   +   2*((a2minc2ovb2 * cos(beta))^2)  +  2 *(  ((b^2 - c^2)/(b^2))  * (cos(alpha))^2  )   - 4*a2plusc2ovb2*cos(alpha)*cos(beta)*cos(gamma)   +   2*((b^2 - a^2)/(b^2))*(cos(gamma)^2);
A2 = 2* A2;
A3 = a2minc2ovb2 * (1 - a2minc2ovb2) * cos(beta)    -   (1 - a2plusc2ovb2) * cos(alpha) * cos(gamma)    +   2 * ((c * cos(alpha)/b)^2) * cos(beta);
A3 = 4 * A3;
A4 = (a2minc2ovb2 -1)^2   - (2 * c * cos(alpha) / b)^2;

%Solve polynomial
%instead of u and v for polynomial, use g and h - i.e., g = s2/s1 and h =
%s3/s1
p = [A4 A3 A2 A1 A0];
h = roots(p);
%choose only real roots - maybe this is not necessary?
h = h(imag(h)==0);
h = real(h);

%%%%%%%%%%%%%%%%%%%%%%%%%%%%%%%%%%%%%%%%%
%%%%%%%%%%%%%Find ray lengths

%For s1, which corresponds to sA. Should end up with 4 solns
%s_A =    (b^2) / (1 + h.^2  +  2*h*cos(beta)  )     ;
%s_A = s_A(s_A~=0);
%s_A = transpose(s_A);
%s_A = s_A.^0.5;


%Find s2, which corresponds to sC.
counter = 1
for i = 1:numel(h)

    s_A = (b^2) / (1 + (h(i)^2) - 2*h(i)*cos(beta));
    s_A = sqrt(s_A);

    G2 = s_A^2;
    G1 = - 2 * (s_A^2) * cos(gamma);
    G0 = (s_A -c)^2;

    g = roots([G2 G1 G0]);
    g = g(imag(g)==0);
    g = real(g);

    %First, solve for s_C, since it only depends on h and s_A:

    for j = 1:numel(g)
        soln(counter, 1) = s_A;
        soln(counter, 3) = s_A * g(j);
        soln(counter, 2) = h(i) * s_A;
        counter = counter +1
    end

end

== matlab function P3P_Grunert/While Iterator Subsystem/Perform P3P and RANSAC on checkerboard/Custom P3P solver (Grunert)/Find ray lengths jingnanshi convention ==
  data: l_AB input; soln output size=[4, 3]; l_BC input; l_AC input; theta input
function soln = fcn(l_AB, l_BC, l_AC, theta)

soln = zeros(4, 3);


%Calculate polynomial coefficients
a = l_AC;
b = l_BC;
c = l_AB;

gamma = theta(1); %theta_AB
alpha = theta(3); %theta_AC
beta = theta(2); %theta_BC


a2minc2ovb2 =  (a^2 - c^2) / b^2 ;
a2plusc2ovb2 =  (a^2 + c^2) / b^2; 


A0 = (1 + a2minc2ovb2)^2   -   4*((a*cos(gamma)/b)^2);
A1 = - a2minc2ovb2 * (1 + a2minc2ovb2) * cos(beta)     +    2 * ((a * cos(gamma) /  b)^2) * cos (beta)     -     (1 - a2plusc2ovb2) * cos(alpha) * cos(gamma);
A1 = 4 * A1;
A2 = a2minc2ovb2^2   -   1   +   2*((a2minc2ovb2 * cos(beta))^2)  +  2 *(  ((b^2 - c^2)/(b^2))  * (cos(alpha))^2  )   - 4*a2plusc2ovb2*cos(alpha)*cos(beta)*cos(gamma)   +   2*((b^2 - a^2)/(b^2))*((cos(gamma))^2);
A2 = 2* A2;
A3 = a2minc2ovb2 * (1 - a2minc2ovb2) * cos(beta)    -   (1 - a2plusc2ovb2) * cos(alpha) * cos(gamma)    +   2 * ((c * cos(alpha)/b)^2) * cos(beta);
A3 = 4 * A3;
A4 = (a2minc2ovb2 -1)^2   - (2 * c * cos(alpha) / b)^2;

%Solve polynomial
%instead of u and v for polynomial, use g and h - i.e., g = s2/s1 and h =
%s3/s1
p = [A4 A3 A2 A1 A0];
h = roots(p);
%choose only real roots - maybe this is not necessary?
h = h(imag(h)==0);
h = real(h);

%%%%%%%%%%%%%%%%%%%%%%%%%%%%%%%%%%%%%%%%%
%%%%%%%%%%%%%Find ray lengths

%For s1, which corresponds to sB. Should end up with 4 solns
%s_A =    (b^2) / (1 + h.^2  +  2*h*cos(beta)  )     ;
%s_A = s_A(s_A~=0);
%s_A = transpose(s_A);
%s_A = s_A.^0.5;


%Find s2, which corresponds to sC.
counter = 1
for i = 1:numel(h)

    s_1 = (b^2) / (1 + (h(i)^2) - 2*h(i)*cos(beta));
    s_1 = sqrt(s_1);

    G2 = s_1^2;
    G1 = - 2 * (s_1^2) * cos(gamma);
    G0 = (s_1^2 -c^2);

    g = roots([G2 G1 G0]);
    g = g(imag(g)==0);
    g = real(g);

    %First, solve for s_C, since it only depends on h and s_A:

    for j = 1:numel(g)
        soln(counter, 1) = s_1 * g(j);
        soln(counter, 3) = s_1 * h(i);
        soln(counter, 2) = s_1; 
        counter = counter +1
    end

end

== matlab function P3P_Grunert/While Iterator Subsystem/Perform P3P and RANSAC on checkerboard/Custom P3P solver (Grunert)/MATLAB Function4 ==
  data: pnts_vectorsCameraCoords input; theta_raysABC_radians output
function theta_raysABC_radians = calcProjectionRayAngles(pnts_vectorsCameraCoords)

A_x_c = pnts_vectorsCameraCoords(:,1);
B_x_c = pnts_vectorsCameraCoords(:,2);
C_x_c = pnts_vectorsCameraCoords(:,3);

%theta_AB = acos(dot(A_x_c, B_x_c));
%theta_BC = acos(dot(B_x_c, C_x_c));
%theta_AC = acos(dot(C_x_c, A_x_c));

%theta_AB = atan2(norm(cross(A_x_c, B_x_c)), dot(A_x_c, B_x_c));
%theta_BC = atan2(norm(cross(B_x_c, C_x_c)), dot(B_x_c, C_x_c));
%theta_AC = atan2(norm(cross(A_x_c, C_x_c)), dot(A_x_c, C_x_c)); 

theta_AB = acos(dot(A_x_c, B_x_c)/(norm(A_x_c)*norm(B_x_c)));
theta_BC = acos(dot(B_x_c, C_x_c)/(norm(B_x_c)*norm(C_x_c)));
theta_AC = acos(dot(A_x_c, C_x_c)/(norm(A_x_c)*norm(C_x_c)));


theta_raysABC_radians = [theta_AB; theta_BC; theta_AC];

== matlab function P3P_Grunert/Subsystem/Custom P3P solver (Grunert)/Calc lengths of triangle sides (world frame) ==
  data: X_ABC_w input; l_AB output; l_BC output; l_AC output
function [l_AB, l_BC, l_AC]= fcn(X_ABC_w)

l_AB = norm(X_ABC_w(:,1)-X_ABC_w(:,2));
l_AC = norm(X_ABC_w(:,1)-X_ABC_w(:,3));
l_BC = norm(X_ABC_w(:,2)-X_ABC_w(:,3));

== matlab function P3P_Grunert/While Iterator Subsystem/Perform P3P and RANSAC on checkerboard/Detect checkerboard corners ==
  data: x_pts_i output size=[60, 2]; I input; checkerSize output size=[1, 2]
function [x_pts_i, checkerSize]= findCheckerboardPnts(I)

%I = imread(fullfile('C:\Users\Alyssa\OneDrive - University of Cape Town\Vision\ESP32-CAM\CamCalibrationPics', '1.jpg'));
Points = detectCheckerboardPoints(I);
[~,checkerSize] = detectCheckerboardPoints(I);
x_pts_i = round(Points);
%checkerSize = Size;
%checkerPoints = imagePoints;

== matlab function P3P_Grunert/While Iterator Subsystem/Perform P3P and RANSAC on checkerboard/Extract best Rte (most inliers) ==
  data: Rte input; bestRt output; bestRt_error output; bestRt_inliers output
function [bestRt, bestRt_error, bestRt_inliers]= fcn(Rte)
%Function looks through 3-dim array Rte to find the Rt that has the highest
%number of inliers. This is output as the "best" Rt


index_bestRte = 0;
mostInliers = 0;

for n=1: size(Rte, 3)

    if Rte(1, 5, n) > mostInliers
        mostInliers = Rte(1, 5, n);
        index_bestRte = n;
    end
end

bestRt = Rte(:, 1:4, index_bestRte);
bestRt_error = Rte(2, 5, index_bestRte);
bestRt_inliers = Rte(1, 5, index_bestRte);

== matlab function P3P_Grunert/While Iterator Subsystem/Perform P3P and RANSAC on checkerboard/For Each Subsystem/Choose best solutiion from iteration ==
  data: Rt input; mostInliers_Rt output size=[3,4]; x_rem_i input; X_rem_w input; mostInliers output; Inlier_threshold input; mostInliers_avgError output; K input
function [mostInliers_Rt, mostInliers, mostInliers_avgError] = fcn(Rt, x_rem_i, X_rem_w, Inlier_threshold, K)
%This function finds the best Rt (transformation matrix) from the current
%RANSAC iteration. Here, "best" means "most inliers". I.e., for each 
%possible Rt out of the P3P solver, each of the remaining detected corners are 
%reprojected (using this Rt). If the reprojection error for a given point
%is below a certain threshold, it is considered an inlier. 
%Out of the 4 possible Rts for each P3P iteration, only that with the
%highest number of iterations will be passed out of this function.

%for each possible solution given by the P3P solver
numTestPts =  size(x_rem_i, 1);
mostInliers = 0;
mostInliers_Rt = zeros(3, 4);
mostInliers_avgError = 0;

for n = 1: size(Rt, 3)

    
    numInliers_n = 0;
    avgError_n = 0;

    %calculate reprojection error 
    for j = 1: numTestPts

        X_j_w = transpose(X_rem_w(j, :));
        x_j_i_real = transpose(x_rem_i(j,:));
        x_j_i_proj = zeros(2, 1);
        x_j_i_proj_homo = zeros(3,1);

        %project point (in homogenous coordinates)
        x_j_i_proj_homo = K * (  (Rt(:, 1:3, n) * X_j_w)  + Rt(:, 4,n)  );

        %Normalise by the 3rd dimension
        x_j_i_proj(1) = x_j_i_proj_homo(1)/x_j_i_proj_homo(3);
        x_j_i_proj(2) = x_j_i_proj_homo(2)/x_j_i_proj_homo(3);

        %calculate reprojection error for current point
        error_j = norm(x_j_i_proj - x_j_i_real);
        avgError_n = avgError_n + error_j;

        %check if an inlier
        if error_j < Inlier_threshold
            numInliers_n = numInliers_n + 1;
        end
    end
    
    %Calculate mean error (could be useful)
    avgError_n = avgError_n / numTestPts;

    %If current Rt achieves more inliers than previous best, then update
    %"best"
    if numInliers_n > mostInliers
        mostInliers = numInliers_n;
        mostInliers_avgError = avgError_n;
        mostInliers_Rt = Rt(:, :, n);
    end
end

== matlab function P3P_Grunert/While Iterator Subsystem/Perform P3P and RANSAC on checkerboard/For Each Subsystem/Create array ==
  data: Rte_n output size=[3,5]; mostInliers_Rt input; mostInliers input; mostInliers_avgError input
function Rte_n = fcn(mostInliers_Rt, mostInliers, mostInliers_avgError)

Rte_n = zeros(3, 5);
Rte_n(:, 1:4) = mostInliers_Rt;
Rte_n(1, 5) = mostInliers;
Rte_n(2, 5) = mostInliers_avgError;
